simulink model "AutopilotControlSystem"  (R2019b)
settings: configuration reference "ctrlConfigSet" (kept outside this file)
undefined symbols (not defined in the file): ap, DiscIntNeverNeededParam, Earth, env, sensors, uav, WGS84
libraries: mbdriLib x74, simulink x12, aerolibtransform2 x5, simulink_need_slupdate x1, aerolibconvert2 x1
(part 2 of 3)

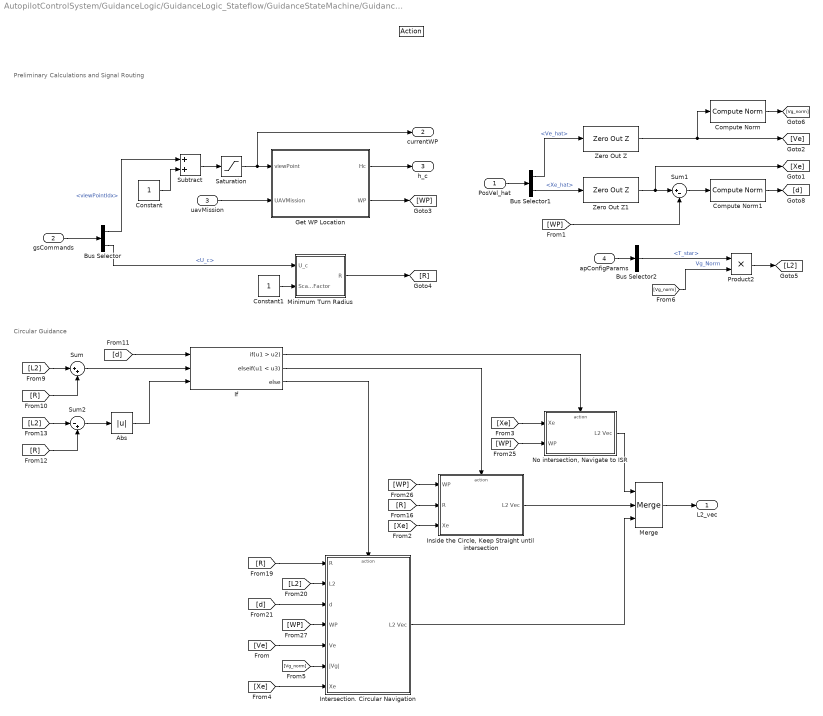
== system AutopilotControlSystem/GuidanceLogic/GuidanceLogic_Stateflow/GuidanceStateMachine/GuidanceLogic.Orbit ==
  note: Preliminary Calculations and Signal Routing
  note: Circular Guidance
  PosVel_hat : Inport
  gsCommands : Inport  Port=2
  uavMission : Inport  Port=3
  apConfigParams : Inport  Port=4
  " " : ActionPort
      settings: CopyFcn=Stateflow.SLINSF.SimulinkMan.removeBlockPreDeleteFcn  PreDeleteFcn=Stateflow.SLINSF.SimulinkMan.unsafePredeleteFcn
  " Compute Norm" : mbdriLib/Utilities/ Compute Norm  SystemSampleTime=-1  Latency=0  AutoFrameSizeCalculation=off
      settings: SourceProductName=Robotics System Toolbox  SourceProductBaseCode=RO
  " Compute Norm1" : mbdriLib/Utilities/ Compute Norm  SystemSampleTime=-1  Latency=0  AutoFrameSizeCalculation=off
      settings: SourceProductName=Robotics System Toolbox  SourceProductBaseCode=RO
  Abs : Abs
  Bus Selector : BusSelector  OutputSignals=viewPointIdx,U_c
  Bus Selector1 : BusSelector  OutputSignals=Ve_hat,Xe_hat
  Bus Selector2 : BusSelector  OutputSignals=T_star
  Constant : Constant  OutDataTypeStr=uint8
      settings: AttributesFormatString=%<Value>
  Constant1 : Constant  OutDataTypeStr=single
      settings: AttributesFormatString=%<Value>
  Get WP Location : Subsystem
  If : If  NumInputs=3  IfExpression=u1 > u2  ElseIfExpressions=u1 < u3
  "Inside the Circle, Keep Straight until intersection" : Subsystem  TreatAsAtomicUnit=on
  Intersection. Circular Navigation : Subsystem  TreatAsAtomicUnit=on
  Merge : Merge  Inputs=3
  Minimum Turn Radius : Subsystem
  "No intersection, Navigate to ISR" : Subsystem  TreatAsAtomicUnit=on
  Product2 : Product
  Saturation : Saturate  UpperLimit=9  LowerLimit=1
      settings: AttributesFormatString=[%<LowerLimit> %<UpperLimit>]
  Subtract : Sum  Inputs=2
  Sum : Sum  Inputs=|++
  Sum1 : Sum  Inputs=|+-
  Sum2 : Sum  Inputs=|-+
  Zero Out Z : mbdriLib/Utilities/Zero Out Z  SystemSampleTime=-1  Latency=0  AutoFrameSizeCalculation=off
      settings: SourceProductName=Robotics System Toolbox  SourceProductBaseCode=RO
  Zero Out Z1 : mbdriLib/Utilities/Zero Out Z  SystemSampleTime=-1  Latency=0  AutoFrameSizeCalculation=off
      settings: SourceProductName=Robotics System Toolbox  SourceProductBaseCode=RO
  L2_vec : Outport  VectorParamsAs1DForOutWhenUnconnected=off
  currentWP : Outport  Port=2  VectorParamsAs1DForOutWhenUnconnected=off
  h_c : Outport  Port=3  VectorParamsAs1DForOutWhenUnconnected=off
  wires:
  [Xe] -> "No intersection, Navigate to ISR"/1(Xe)
  " Compute Norm1"/1 -> [d]
  [WP] -> Intersection. Circular Navigation/4(WP)
  Abs/1 -> If/3
  [Xe] -> Intersection. Circular Navigation/7(Xe)
  Intersection. Circular Navigation/1(L2 Vec) -> Merge/3
  Bus Selector/1 -> Subtract/1  "<viewPointIdx>"
  If/2 -> "Inside the Circle, Keep Straight until intersection"/Action
  [R] -> Intersection. Circular Navigation/1(R)
  "No intersection, Navigate to ISR"/1(L2 Vec) -> Merge/1
  [R] -> Sum2/2
  If/3 -> Intersection. Circular Navigation/Action
  [L2] -> Sum2/1
  "Inside the Circle, Keep Straight until intersection"/1(L2 Vec) -> Merge/2
  uavMission/1 -> Get WP Location/2(UAVMission)
  [Vg_norm] -> Intersection. Circular Navigation/6(|Vg|)
  [Xe] -> "Inside the Circle, Keep Straight until intersection"/3(Xe)
  [WP] -> "No intersection, Navigate to ISR"/2(WP)
  [WP] -> "Inside the Circle, Keep Straight until intersection"/1(WP)
  Get WP Location/2(WP) -> [WP]
  [L2] -> Sum/1
  Subtract/1 -> Saturation/1
  Saturation/1 -> currentWP/1, Get WP Location/1(viewPoint)
  Merge/1 -> L2_vec/1
  Constant/1 -> Subtract/2
  Sum2/1 -> Abs/1
  If/1 -> "No intersection, Navigate to ISR"/Action
  [WP] -> Sum1/2
  [R] -> Sum/2
  [L2] -> Intersection. Circular Navigation/2(L2)
  Sum/1 -> If/2
  [Ve] -> Intersection. Circular Navigation/5(Ve)
  [d] -> If/1
  [R] -> "Inside the Circle, Keep Straight until intersection"/2(R)
  [d] -> Intersection. Circular Navigation/3(d)
  Get WP Location/1(Hc) -> h_c/1
  gsCommands/1 -> Bus Selector/1
  PosVel_hat/1 -> Bus Selector1/1
  Bus Selector1/1 -> Zero Out Z/1  "<Ve_hat>"
  Sum1/1 -> " Compute Norm1"/1
  Zero Out Z/1 -> " Compute Norm"/1, [Ve]
  " Compute Norm"/1 -> [Vg_norm]
  apConfigParams/1 -> Bus Selector2/1
  [Vg_norm] -> Product2/2  "Vg_Norm"
  Product2/1 -> [L2]
  Bus Selector2/1 -> Product2/1  "<T_star>"
  Bus Selector/2 -> Minimum Turn Radius/1(U_c)  "<U_c>"
  Constant1/1 -> Minimum Turn Radius/2(Scale Factor)
  Minimum Turn Radius/1(R) -> [R]
  Zero Out Z1/1 -> Sum1/1, [Xe]
  Bus Selector1/2 -> Zero Out Z1/1  "<Xe_hat>"

== system AutopilotControlSystem/GuidanceLogic/GuidanceLogic_Stateflow/GuidanceStateMachine/GuidanceLogic.RTB ==
  PosVel_hat : Inport
  gsCommands : Inport  Port=2
  uavMission : Inport  Port=3
  " " : ActionPort
      settings: CopyFcn=Stateflow.SLINSF.SimulinkMan.removeBlockPreDeleteFcn  PreDeleteFcn=Stateflow.SLINSF.SimulinkMan.unsafePredeleteFcn
  Bus Selector : BusSelector  OutputSignals=h_c_midLevel,followMobile,MobileLocation
  Bus Selector1 : BusSelector  OutputSignals=Xe_hat
  Constant : Constant  Value=[0 0 0]  OutDataTypeStr=single
      settings: AttributesFormatString=%<Value>
  Get Mobile Location : Subsystem
  RTB1 : Constant  OutDataTypeStr=uint8
      settings: AttributesFormatString=%<Value>
  RTB2 : Constant  OutDataTypeStr=single
      settings: AttributesFormatString=%<Value>
  Simple Predictor : Subsystem
  Slider Gain : simulink/Math Operations/Slider Gain  gain=3  low=1  high=20
  Subtract : Sum  Inputs=+-
  Switch : Switch  Criteria=u2 > Threshold
  Zero Out Z : mbdriLib/Utilities/Zero Out Z  SystemSampleTime=-1  Latency=0  AutoFrameSizeCalculation=off
      settings: SourceProductName=Robotics System Toolbox  SourceProductBaseCode=RO
  L2_vec : Outport  VectorParamsAs1DForOutWhenUnconnected=off
  h_c : Outport  Port=2  VectorParamsAs1DForOutWhenUnconnected=off
  currentWP : Outport  Port=3  VectorParamsAs1DForOutWhenUnconnected=off
  wires:
  gsCommands/1 -> Bus Selector/1
  Bus Selector/3 -> Get Mobile Location/1(Mobile Loc)  "<MobileLocation>"
  Bus Selector/2 -> Get Mobile Location/Enable, Switch/2  "<followMobile>"
  Bus Selector/1 -> h_c/1  "<h_c_midLevel>"
  Simple Predictor/1(Predicted Bp) -> L2_vec/1
  RTB1/1 -> currentWP/1
  PosVel_hat/1 -> Bus Selector1/1
  Bus Selector1/1 -> Zero Out Z/1  "<Xe_hat>"
  Zero Out Z/1 -> Subtract/2
  uavMission/1 -> Get Mobile Location/2(UAVMission)
  Slider Gain/1 -> Simple Predictor/2(Prediction Gain)
  RTB2/1 -> Slider Gain/1
  Switch/1 -> Subtract/1
  Subtract/1 -> Simple Predictor/1(Base Point)
  Get Mobile Location/1(MobileLTP) -> Switch/1
  Constant/1 -> Switch/3

== system AutopilotControlSystem/GuidanceLogic/GuidanceLogic_Stateflow/GuidanceStateMachine/GuidanceLogic.WP ==
  note: Curry, R., Lizarraga, M., Elkaim, G., Mairs, B., “L2+, an Improved Line of Sight Guidance Law for UAVs”
      | American Control Conference, ACC13, Washington D.C., 17-19 June 2013
  PosVel_hat : Inport
  gsCommands : Inport  Port=2
  uavMission : Inport  Port=3
  apConfigParams : Inport  Port=4
  " " : ActionPort
      settings: CopyFcn=Stateflow.SLINSF.SimulinkMan.removeBlockPreDeleteFcn  PreDeleteFcn=Stateflow.SLINSF.SimulinkMan.unsafePredeleteFcn
  Bus Selector : BusSelector  OutputSignals=isManualModeOn
  Bus Selector1 : BusSelector  OutputSignals=Ve_hat,Xe_hat
  Bus Selector2 : BusSelector  OutputSignals=T_star,turnLead
  Compute Distance to WP : Subsystem
  Compute L2 Vector : Subsystem
  Compute Vg_norm : Subsystem
  Delay : Delay  DelayLength=1  InitialCondition=1000
  Display : Display
  Get Next Waypoint : Subsystem
  Logical Operator : Logic  Operator=NOT  AllPortsSameDT=off  OutDataTypeStr=boolean
  MATLAB Function : MATLAB Function  TreatAsAtomicUnit=on
  Product1 : Product  OutDataTypeStr=single  RndMeth=Zero
  Product2 : Product
  Recent Enable : Subsystem
  Subtract : Sum  Inputs=+-
  Wp Switching Logic : mbdriLib/Guidance/Wp Switching Logic  SystemSampleTime=-1  Latency=0  AutoFrameSizeCalculation=off
      settings: SourceProductName=Robotics System Toolbox  SourceProductBaseCode=RO
  L2_vec : Outport  VectorParamsAs1DForOutWhenUnconnected=off
  currentWP : Outport  Port=2  VectorParamsAs1DForOutWhenUnconnected=off
  h_c : Outport  Port=3  VectorParamsAs1DForOutWhenUnconnected=off
  wires:
  Recent Enable/1(WPEnable) -> Wp Switching Logic/3
  uavMission/1 -> MATLAB Function/1(u), Get Next Waypoint/1(UAVMission)
  Wp Switching Logic/1 -> Get Next Waypoint/2(From WP)
  Subtract/1 -> Delay/1
  Delay/1 -> Wp Switching Logic/1
  Compute Distance to WP/1(Dist2WpT) -> Subtract/1, Compute L2 Vector/1(Dist2WP)
  Product1/1 -> Subtract/2  "turnLeadDistance"
  [Xe] -> Compute L2 Vector/5(Xe)
  Get Next Waypoint/1(H_c) -> h_c/1
  Compute L2 Vector/1(L2Vec) -> L2_vec/1
  Get Next Waypoint/3(T) -> Compute L2 Vector/3(T), Compute Distance to WP/3(T)
  Product2/1 -> Get Next Waypoint/4(L2), Compute L2 Vector/6(L2)
  Get Next Waypoint/2(WPT) -> Compute L2 Vector/2(WPT), Compute Distance to WP/2(WPT)
  Get Next Waypoint/4(N) -> Compute L2 Vector/4(N)
  MATLAB Function/1(maxWp) -> Wp Switching Logic/2
  Wp Switching Logic/2 -> currentWP/1, Get Next Waypoint/3(To WP)
  gsCommands/1 -> Bus Selector/1
  Logical Operator/1 -> Recent Enable/1(WP Fly)
  Bus Selector/1 -> Logical Operator/1  "<isManualModeOn>"
  PosVel_hat/1 -> Bus Selector1/1
  Bus Selector1/2 -> Display/1, [Xe], Compute Distance to WP/1(Xe)  "<Xe_hat>"
  [Vg_norm] -> Product2/2  "Vg_Norm"
  apConfigParams/1 -> Bus Selector2/1
  Compute Vg_norm/1(|Vg|) -> [Vg_norm], Product1/2
  Bus Selector1/1 -> Compute Vg_norm/1(<Ve_hat>)  "<Ve_hat>"
  [turnLead] -> Product1/1
  Bus Selector2/1 -> Product2/1  "<T_star>"
  Bus Selector2/2 -> [turnLead]  "<turnLead>"

== system AutopilotControlSystem/InnerLoopAutopilot/Latch Trim Conditions/Latch Control Surfaces Trim from any mode ==
  ctrlSurfaces : Inport
  Trigger : TriggerPort  TriggerType=falling  VariantControl=Variant
  Trim : Outport  VectorParamsAs1DForOutWhenUnconnected=off
  wires:
  ctrlSurfaces/1 -> Trim/1

== system AutopilotControlSystem/InnerLoopAutopilot/Longitudinal Channel/Compute Feed Forward ==
  dEFFGain : Inport
  SensorData : Inport  Port=2
  1D Discrete Filter : mbdriLib/Filtering/1D Discrete Filter  bw=10  TSample=ap.apSampleTime
      settings: AttributesFormatString=Fc = 10  SourceProductName=Robotics System Toolbox  SourceProductBaseCode=RO
  Add5 : Sum  Inputs=+-  OutDataTypeStr=single
  Bus Selector : BusSelector  OutputSignals=Euler
  Constant2 : Constant  OutDataTypeStr=single
      settings: AttributesFormatString=%<Value>
  Constant4 : Constant  OutDataTypeStr=single
      settings: AttributesFormatString=%<Value>
  Product : Product  Inputs=*/  RndMeth=Zero
  Product1 : Product  RndMeth=Zero
  Selector : Selector  InputPortWidth=3  IndexOptions=Index vector (dialog)  Indices=[1]  OutputSizes=1
  Trigonometric Function : Trigonometry  Operator=cos
  "[-60 60]" : Saturate  UpperLimit=60  LowerLimit=-60
      settings: AttributesFormatString="[%<LowerLimit>  %<UpperLimit>]"
  FF : Outport  VectorParamsAs1DForOutWhenUnconnected=off
  wires:
  Selector/1 -> 1D Discrete Filter/1
  Product/1 -> Add5/1
  Constant4/1 -> Product/1
  1D Discrete Filter/1 -> "[-60 60]"/1
  Trigonometric Function/1 -> Product/2
  Constant2/1 -> Add5/2
  Product1/1 -> FF/1
  Add5/1 -> Product1/2
  "[-60 60]"/1 -> Trigonometric Function/1
  Bus Selector/1 -> Selector/1  "<Euler>"
  dEFFGain/1 -> Product1/1
  SensorData/1 -> Bus Selector/1

== system AutopilotControlSystem/InnerLoopAutopilot/Longitudinal Channel/Height Error to Pitch Command [PI] ==
  Error : Inport
  Reset : Inport  Port=2
  PIDGains : Inport  Port=3
  Demux : Demux  Outputs=3
  PID Controller : simulink/Continuous/PID Controller  Controller=PI  Form=Parallel  TimeDomain=Discrete-time  SampleTime=ap.apSampleTime  IntegratorMethod=Trapezoidal  FilterMethod=Forward Euler  ControllerParametersSource=external  P=1  I=1  D=0  UseFilter=on  N=100  TunerSelectOption=Transfer Function Based (PID Tuner App)  InitialConditionSource=internal  InitialConditionForIntegrator=0  InitialConditionForFilter=0  DifferentiatorICPrevScaledInput=0  ExternalReset=level  TrackingMode=off  Kt=1  LimitOutput=on  UpperSaturationLimit=ap.control.the_cLimit  LowerSaturationLimit=-ap.control.the_cLimit  LinearizeAsGain=on  AntiWindupMode=clamping  Kb=1  POutMin=[]  POutMax=[]  IOutMin=[]  IOutMax=[]  DOutMin=[]  DOutMax=[]  NOutMin=[]  NOutMax=[]  SumOutMin=[]  SumOutMax=[]  SaturationOutMin=[]  SaturationOutMax=[]  PParamMin=[]  PParamMax=[]  IParamMin=[]  IParamMax=[]  DParamMin=[]  DParamMax=[]  NParamMin=[]  NParamMax=[]  KbParamMin=[]  KbParamMax=[]  KtParamMin=[]  KtParamMax=[]  KbOutMin=[]  KbOutMax=[]  KtOutMin=[]  KtOutMax=[]  IntegratorOutMin=[]  IntegratorOutMax=[]  FilterOutMin=[]  FilterOutMax=[]  SumI1OutMin=[]  SumI1OutMax=[]  SumI2OutMin=[]  SumI2OutMax=[]  SumI3OutMin=[]  SumI3OutMax=[]  SumI4OutMin=[]  SumI4OutMax=[]  SumDOutMin=[]  SumDOutMax=[]  DifferentiatorOutMin=[]  DifferentiatorOutMax=[]  FilterDiffOutCoefMin=[]  FilterDiffOutCoefMax=[]  ReciprocalOutMin=[]  ReciprocalOutMax=[]  SumDenOutMin=[]  SumDenOutMax=[]  SumNumOutMin=[]  SumNumOutMax=[]  DivideOutMin=[]  DivideOutMax=[]  IntegratorContinuousStateAttributes=''  IntegratorStateMustResolveToSignalObject=off  IntegratorRTWStateStorageClass=Auto  FilterContinuousStateAttributes=''  FilterStateMustResolveToSignalObject=off  FilterRTWStateStorageClass=Auto  ParallelPVariant=ExternalParameters  IdealPVariant=Disabled  IVariant=ExternalParameters  DVariant=Disabled  IntegratorVariant=Discrete  SatVariant=Enabled  AWVariant=DiscClampingParallel  PCopyVariant=Disabled  TRVariant=Disabled  FdbkBlocksVariant=Feedback  IdealPFdbkVariant=Passthrough  SatFdbkVariant=Passthrough  DerivativeFilterVariant=Disabled  NVariant=Disabled  NCopyVariant=Disabled_SignalSpec  FilterICVariant=Disabled  IntegratorICVariant=InternalICs  ExternalResetVariant=ExternalReset  TRSumVariant=Passthrough  SumFdbkVariant=Enabled  SumVariant=Sum_PI
  Terminator : Terminator
  Output : Outport  VectorParamsAs1DForOutWhenUnconnected=off
  wires:
  Demux/3 -> Terminator/1
  Error/1 -> PID Controller/1
  PIDGains/1 -> Demux/1
  Demux/1 -> PID Controller/2
  Demux/2 -> PID Controller/3
  Reset/1 -> PID Controller/4
  PID Controller/1 -> Output/1

== system AutopilotControlSystem/InnerLoopAutopilot/Longitudinal Channel/Rate Limiter Dynamic with External IC and Autoreset for Change in IC ==
  note: Y(k)
  note: U(k)
  up : Inport
  u : Inport  Port=2
  IC : Inport  Port=3
  lo : Inport  Port=4
  Capture/Reset IC : Subsystem
  Difference Inputs1 : Sum  Description=Add in CPU  DisableCoverage=on  Inputs=+-  OutDataTypeStr=Inherit: Inherit via back propagation
  Difference Inputs2 : Sum  Description=Add in CPU  OutDataTypeStr=Inherit: Inherit via back propagation
  FixPt Data Type Duplicate : DataTypeDuplicate  DisableCoverage=on  NumInputPorts=7
  Saturation Dynamic : simulink/Discontinuities/Saturation Dynamic  OutMin=[]  OutMax=[]  OutDataTypeStr=Inherit: Same as second input  OutDataType=fixdt(1, 16)  OutScaling=2^-10  DoSatur=off
  delta fall limit : Product  DisableCoverage=on  Inputs=**  OutDataTypeStr=Inherit: Inherit via back propagation  SaturateOnIntegerOverflow=on
  delta rise limit : Product  DisableCoverage=on  Inputs=**  OutDataTypeStr=Inherit: Inherit via back propagation  SaturateOnIntegerOverflow=on
  sample time : SampleTimeMath  DisableCoverage=on  TsampMathOp=Ts Only  weightValue=1
  Y : Outport  VectorParamsAs1DForOutWhenUnconnected=off
  wires:
  sample time/1 -> delta fall limit/2, delta rise limit/2
  lo/1 -> delta fall limit/1
  delta rise limit/1 -> FixPt Data Type Duplicate/6, Saturation Dynamic/1
  up/1 -> delta rise limit/1
  Difference Inputs2/1 -> FixPt Data Type Duplicate/1, Capture/Reset IC/1(Y(k)), Y/1
  Saturation Dynamic/1 -> Difference Inputs2/1, FixPt Data Type Duplicate/7
  delta fall limit/1 -> FixPt Data Type Duplicate/3, Saturation Dynamic/3
  u/1 -> Difference Inputs1/1, FixPt Data Type Duplicate/5, sample time/1
  Difference Inputs1/1 -> FixPt Data Type Duplicate/4, Saturation Dynamic/2  "( U(k) - Y(k-1) )"
  Capture/Reset IC/1(Y(k-1)) -> Difference Inputs2/2, FixPt Data Type Duplicate/2, Difference Inputs1/2
  IC/1 -> Capture/Reset IC/2(IC)

== system AutopilotControlSystem/Navigation Filter/Get Vn Ve/Subsystem5 ==
  u : Inport
  Trigonometric Function : Trigonometry
  Trigonometric Function1 : Trigonometry  Operator=cos
  sin(u) : Outport  VectorParamsAs1DForOutWhenUnconnected=off
  cos(u) : Outport  Port=2  VectorParamsAs1DForOutWhenUnconnected=off
  wires:
  u/1 -> Trigonometric Function/1, Trigonometric Function1/1
  Trigonometric Function/1 -> sin(u)/1
  Trigonometric Function1/1 -> cos(u)/1

== system AutopilotControlSystem/Navigation Filter/Position&Velocity Filter/CompRateOnly ==
  LoPass : Inport
  Gain : Gain  Gain=omega
      settings: AttributesFormatString=%<Gain>
  Sum1 : Sum  Inputs=|+-
  Unit Delay : UnitDelay  SampleTime=T  HasFrameUpgradeWarning=on
  ZPK 1D Discrete Filter : mbdriLib/Filtering/ZPK 1D Discrete Filter  zval=[]  pval=[0]  kval=1  TSample=0.01
      settings: SourceProductName=Robotics System Toolbox  SourceProductBaseCode=RO
  Rate_hat : Outport  VectorParamsAs1DForOutWhenUnconnected=off
  wires:
  Unit Delay/1 -> Sum1/2
  LoPass/1 -> Sum1/1
  Sum1/1 -> Gain/1
  Gain/1 -> ZPK 1D Discrete Filter/1, Rate_hat/1
  ZPK 1D Discrete Filter/1 -> Unit Delay/1

== system AutopilotControlSystem/Navigation Filter/Position&Velocity Filter/Deriv  ==
  y : Inport
  Gain2 : Gain  Gain=[ 1/(5*ap.apSampleTime) ]
      settings: AttributesFormatString=%<Gain>
  Integer Delay1 : Delay  DelayLength=5  InitialCondition=0  SampleTime=ap.apSampleTime
  Sum5 : Sum  Inputs=-+|
  ydot : Outport  VectorParamsAs1DForOutWhenUnconnected=off
  wires:
  Gain2/1 -> ydot/1
  y/1 -> Integer Delay1/1, Sum5/2
  Integer Delay1/1 -> Sum5/1
  Sum5/1 -> Gain2/1

== system AutopilotControlSystem/Navigation Filter/Position&Velocity Filter/VN Ve Filter ==
  Vn : Inport
  Ve : Inport  Port=2
  New GPS : Inport  Port=3
  Enable : EnablePort
  Constant : Constant  Value=ap.apSampleTime
      settings: AttributesFormatString=%<Value>
  RateAid for GPS : mbdriLib/Filtering/RateAid for GPS  SystemSampleTime=-1  Latency=0  AutoFrameSizeCalculation=off
      settings: SourceProductName=Robotics System Toolbox  SourceProductBaseCode=RO
  RateAid for GPS1 : mbdriLib/Filtering/RateAid for GPS  SystemSampleTime=-1  Latency=0  AutoFrameSizeCalculation=off
      settings: SourceProductName=Robotics System Toolbox  SourceProductBaseCode=RO
  Vn_fil : Outport  OutputWhenDisabled=reset  InitialOutput=0  VectorParamsAs1DForOutWhenUnconnected=off
  Ve_fil : Outport  Port=2  OutputWhenDisabled=reset  InitialOutput=0  VectorParamsAs1DForOutWhenUnconnected=off
  wires:
  Constant/1 -> RateAid for GPS1/3, RateAid for GPS/3
  New GPS/1 -> RateAid for GPS/2, RateAid for GPS1/2
  Vn/1 -> RateAid for GPS/1
  Ve/1 -> RateAid for GPS1/1
  RateAid for GPS/1 -> Vn_fil/1
  RateAid for GPS1/1 -> Ve_fil/1

== system AutopilotControlSystem/Navigation Filter/Position&Velocity Filter/Z Comp Filter ==
  note: Lizarraga, Mariano I. Autonomous landing system for a UAV . Master's Thesis. Monterey California. Naval Postgraduate School, 2004.
  Az : Inport
  Baro Alt : Inport  Port=2
  Xe_z_ic : Inport  Port=3
  Constant : Constant  Value=env.ISA_g  OutDataTypeStr=single
      settings: AttributesFormatString=%<Value>
  Discrete-Time Integrator : DiscreteIntegrator  gainval=1  SampleTime=-1  ICPrevOutput=DiscIntNeverNeededParam  ICPrevScaledInput=DiscIntNeverNeededParam
  Discrete-Time Integrator1 : DiscreteIntegrator  gainval=1  SampleTime=-1  ICPrevOutput=DiscIntNeverNeededParam  ICPrevScaledInput=DiscIntNeverNeededParam
  Discrete-Time Integrator2 : DiscreteIntegrator  gainval=1  InitialConditionSource=external  SampleTime=-1  ICPrevOutput=DiscIntNeverNeededParam  ICPrevScaledInput=DiscIntNeverNeededParam
  Gain : Gain  Gain=21  OutDataTypeStr=single
      settings: AttributesFormatString=%<Gain>
  Gain1 : Gain  Gain=9  OutDataTypeStr=single
      settings: AttributesFormatString=%<Gain>
  Gain2 : Gain  Gain=15  OutDataTypeStr=single
      settings: AttributesFormatString=%<Gain>
  Sum : Sum  Inputs=|++
  Sum1 : Sum  Inputs=+++
  Sum2 : Sum  Inputs=-+|
  Sum3 : Sum  Inputs=|++
  Xe_Z_hat : Outport  VectorParamsAs1DForOutWhenUnconnected=off
  wires:
  Discrete-Time Integrator2/1 -> Sum2/1, Xe_Z_hat/1
  Gain2/1 -> Sum3/2
  Gain1/1 -> Discrete-Time Integrator/1
  Gain/1 -> Sum1/3
  Sum2/1 -> Gain2/1, Gain/1, Gain1/1
  Sum3/1 -> Discrete-Time Integrator2/1
  Discrete-Time Integrator1/1 -> Sum3/1
  Baro Alt/1 -> Sum2/2
  Xe_z_ic/1 -> Discrete-Time Integrator2/2
  Sum1/1 -> Discrete-Time Integrator1/1
  Sum/1 -> Sum1/1
  Discrete-Time Integrator/1 -> Sum1/2
  Constant/1 -> Sum/2
  Az/1 -> Sum/1

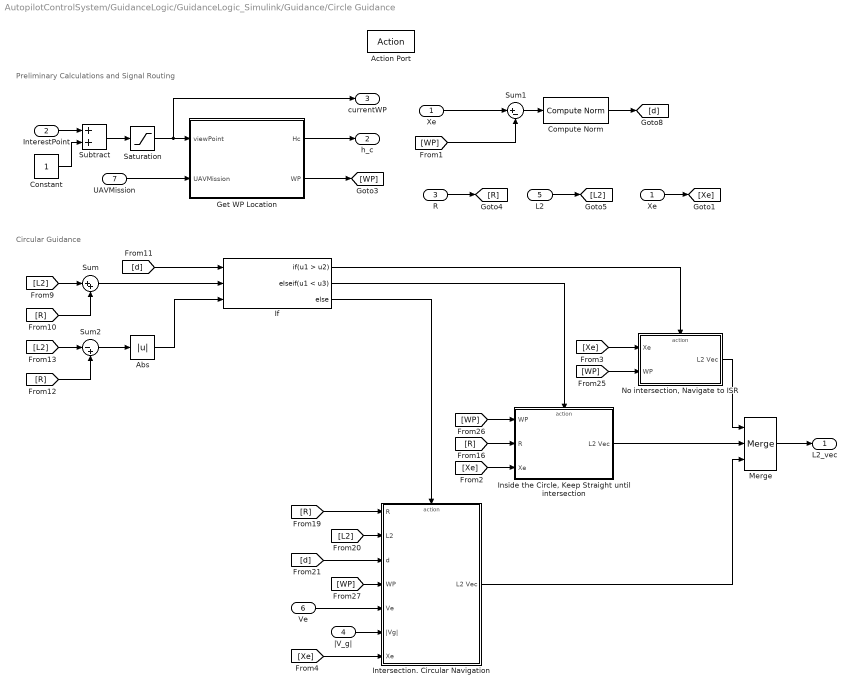
== system AutopilotControlSystem/GuidanceLogic/GuidanceLogic_Simulink/Guidance/Circle Guidance ==
  note: Preliminary Calculations and Signal Routing
  note: Circular Guidance
  Xe : Inport
  InterestPoint : Inport  Port=2
  R : Inport  Port=3
  |V_g| : Inport  Port=4
  L2 : Inport  Port=5
  Ve : Inport  Port=6
  UAVMission : Inport  Port=7
  Action Port : ActionPort  ActionPortLabel=elseif { }
  " Compute Norm" : mbdriLib/Utilities/ Compute Norm
      settings: SourceProductName=Robotics System Toolbox  SourceProductBaseCode=RO
  Abs : Abs
  Constant : Constant  OutDataTypeStr=uint8
      settings: AttributesFormatString=%<Value>
  Get WP Location : Subsystem
  If : If  NumInputs=3  IfExpression=u1 > u2  ElseIfExpressions=u1 < u3
  "Inside the Circle, Keep Straight until intersection" : Subsystem  TreatAsAtomicUnit=on
  Intersection. Circular Navigation : Subsystem  TreatAsAtomicUnit=on
  Merge : Merge  Inputs=3
  "No intersection, Navigate to ISR" : Subsystem  TreatAsAtomicUnit=on
  Saturation : Saturate  UpperLimit=9  LowerLimit=1
      settings: AttributesFormatString=[%<LowerLimit> %<UpperLimit>]
  Subtract : Sum  Inputs=2
  Sum : Sum  Inputs=|++
  Sum1 : Sum  Inputs=|+-
  Sum2 : Sum  Inputs=|-+
  "Xe   " : InportShadow
  L2_vec : Outport  VectorParamsAs1DForOutWhenUnconnected=off
  h_c : Outport  Port=2  VectorParamsAs1DForOutWhenUnconnected=off
  currentWP : Outport  Port=3  VectorParamsAs1DForOutWhenUnconnected=off
  wires:
  Saturation/1 -> Get WP Location/1(viewPoint), currentWP/1
  InterestPoint/1 -> Subtract/1
  Subtract/1 -> Saturation/1
  Constant/1 -> Subtract/2
  [Xe] -> "No intersection, Navigate to ISR"/1(Xe)
  [Xe] -> "Inside the Circle, Keep Straight until intersection"/3(Xe)
  Xe/1 -> [Xe]
  Intersection. Circular Navigation/1(L2 Vec) -> Merge/3
  "Inside the Circle, Keep Straight until intersection"/1(L2 Vec) -> Merge/2
  "No intersection, Navigate to ISR"/1(L2 Vec) -> Merge/1
  UAVMission/1 -> Get WP Location/2(UAVMission)
  R/1 -> [R]
  Get WP Location/2(WP) -> [WP]
  L2/1 -> [L2]
  [L2] -> Sum/1
  [R] -> Sum/2
  "Xe   "/1 -> Sum1/1
  [WP] -> Sum1/2
  Sum1/1 -> " Compute Norm"/1
  " Compute Norm"/1 -> [d]
  [d] -> If/1
  Sum/1 -> If/2
  [L2] -> Sum2/1
  [R] -> Sum2/2
  Sum2/1 -> Abs/1
  Abs/1 -> If/3
  Merge/1 -> L2_vec/1
  If/1 -> "No intersection, Navigate to ISR"/Action
  If/2 -> "Inside the Circle, Keep Straight until intersection"/Action
  If/3 -> Intersection. Circular Navigation/Action
  [WP] -> "No intersection, Navigate to ISR"/2(WP)
  [WP] -> "Inside the Circle, Keep Straight until intersection"/1(WP)
  [R] -> "Inside the Circle, Keep Straight until intersection"/2(R)
  [R] -> Intersection. Circular Navigation/1(R)
  [L2] -> Intersection. Circular Navigation/2(L2)
  [d] -> Intersection. Circular Navigation/3(d)
  [WP] -> Intersection. Circular Navigation/4(WP)
  Ve/1 -> Intersection. Circular Navigation/5(Ve)
  |V_g|/1 -> Intersection. Circular Navigation/6(|Vg|)
  Get WP Location/1(Hc) -> h_c/1
  [Xe] -> Intersection. Circular Navigation/7(Xe)

== system AutopilotControlSystem/GuidanceLogic/GuidanceLogic_Simulink/Guidance/Mid Level Direct Commands ==
  psiDot_c_ml : Inport
  h_c_midLvl : Inport  Port=2
  U_m : Inport  Port=3
  Action Port : ActionPort  ActionPortLabel=elseif { }
  RTB1 : Constant  Value=0  OutDataTypeStr=uint8
      settings: AttributesFormatString=%<Value>
  psi_dot to phi : mbdriLib/Angles and Units/psi_dot to phi
      settings: SourceProductName=Robotics System Toolbox  SourceProductBaseCode=RO
  phi_c_ml : Outport  VectorParamsAs1DForOutWhenUnconnected=off
  h_c : Outport  Port=2  VectorParamsAs1DForOutWhenUnconnected=off
  currentWP : Outport  Port=3  VectorParamsAs1DForOutWhenUnconnected=off
  wires:
  RTB1/1 -> currentWP/1
  psi_dot to phi/1 -> phi_c_ml/1
  psiDot_c_ml/1 -> psi_dot to phi/1
  U_m/1 -> psi_dot to phi/2
  h_c_midLvl/1 -> h_c/1

== system AutopilotControlSystem/GuidanceLogic/GuidanceLogic_Simulink/Guidance/Minimum Turn Radius ==
  U_c : Inport
  Scale Factor : Inport  Port=2
  Constant1 : Constant  Value=ap.guidance.maxAcc  OutDataTypeStr=single
      settings: AttributesFormatString=%<Value>
  IC : InitialCondition  Value=1.5
  Math Function : Math  Operator=square  SaturateOnIntegerOverflow=on
  Product2 : Product  RndMeth=Zero
  Product3 : Product  Inputs=*/  RndMeth=Zero
  "[1.5 10]" : Saturate  UpperLimit=10  LowerLimit=1.5
      settings: AttributesFormatString="[%<LowerLimit>  %<UpperLimit>]"
  R : Outport  VectorParamsAs1DForOutWhenUnconnected=off
  wires:
  IC/1 -> "[1.5 10]"/1
  "[1.5 10]"/1 -> Product2/1
  Product3/1 -> R/1
  Scale Factor/1 -> IC/1
  Math Function/1 -> Product2/2
  Constant1/1 -> Product3/2
  Product2/1 -> Product3/1
  U_c/1 -> Math Function/1

== system AutopilotControlSystem/GuidanceLogic/GuidanceLogic_Simulink/Guidance/RTB//Follow Mobile Guidance ==
  Mobile Location : Inport
  Follow Mobile? : Inport  Port=2
  MidLvl h_c : Inport  Port=3
  Puav : Inport  Port=4
  UAVMission : Inport  Port=5
  Action Port : ActionPort  ActionPortLabel=if { }
  Constant : Constant  Value=[0 0 0]  OutDataTypeStr=single
      settings: AttributesFormatString=%<Value>
  Get Mobile Location : Subsystem
  RTB1 : Constant  OutDataTypeStr=uint8
      settings: AttributesFormatString=%<Value>
  RTB2 : Constant  OutDataTypeStr=single
      settings: AttributesFormatString=%<Value>
  Simple Predictor : Subsystem
  Slider Gain : simulink/Math Operations/Slider Gain  gain=3  low=1  high=20
  Subtract : Sum  Inputs=+-
  Switch : Switch  Criteria=u2 > Threshold
  L2_vec : Outport  VectorParamsAs1DForOutWhenUnconnected=off
  h_c : Outport  Port=2  VectorParamsAs1DForOutWhenUnconnected=off
  currentWP : Outport  Port=3  VectorParamsAs1DForOutWhenUnconnected=off
  wires:
  RTB1/1 -> currentWP/1
  UAVMission/1 -> Get Mobile Location/2(UAVMission)
  Slider Gain/1 -> Simple Predictor/2(Prediction Gain)
  RTB2/1 -> Slider Gain/1
  MidLvl h_c/1 -> h_c/1
  Switch/1 -> Subtract/1
  Puav/1 -> Subtract/2
  Subtract/1 -> Simple Predictor/1(Base Point)
  Simple Predictor/1(Predicted Bp) -> L2_vec/1
  Mobile Location/1 -> Get Mobile Location/1(Mobile Loc)
  Follow Mobile?/1 -> Get Mobile Location/Enable, Switch/2
  Get Mobile Location/1(MobileLTP) -> Switch/1
  Constant/1 -> Switch/3

== system AutopilotControlSystem/GuidanceLogic/GuidanceLogic_Simulink/Guidance/Recent Enable ==
  WP Fly : Inport
  IC1 : InitialCondition  Value=0
  Subsystem : Subsystem
  WPEnable : Outport  VectorParamsAs1DForOutWhenUnconnected=off
  wires:
  WP Fly/1 -> IC1/1
  Subsystem/1(Just Enab) -> WPEnable/1
  IC1/1 -> Subsystem/1(WP Fly)

== system AutopilotControlSystem/GuidanceLogic/GuidanceLogic_Simulink/Guidance/WP Guidance ==
  note: Curry, R., Lizarraga, M., Elkaim, G., Mairs, B., “L2+, an Improved Line of Sight Guidance Law for UAVs”
      | American Control Conference, ACC13, Washington D.C., 17-19 June 2013
  UAVMission : Inport
  Xe : Inport  Port=2
  L2 : Inport  Port=3
  MaxWP : Inport  Port=4
  turnLeadTime : Inport  Port=5
  V_g : Inport  Port=6
  WpEnable : Inport  Port=7
  Action Port : ActionPort  ActionPortLabel=elseif { }
  Compute Distance to WP : Subsystem
  Compute L2 Vector : Subsystem
  Delay : Delay  DelayLength=1  InitialCondition=1000
  Get Next Waypoint : Subsystem
  Product1 : Product  OutDataTypeStr=single  RndMeth=Zero
  Subtract : Sum  Inputs=+-
  Wp Switching Logic : mbdriLib/Guidance/Wp Switching Logic  SystemSampleTime=-1
      settings: SourceProductName=Robotics System Toolbox  SourceProductBaseCode=RO
  L2Vec : Outport  VectorParamsAs1DForOutWhenUnconnected=off
  h_c : Outport  Port=2  VectorParamsAs1DForOutWhenUnconnected=off
  currentWP : Outport  Port=3  VectorParamsAs1DForOutWhenUnconnected=off
  wires:
  Get Next Waypoint/1(H_c) -> h_c/1
  WpEnable/1 -> Wp Switching Logic/3
  Product1/1 -> Subtract/2  "turnLeadDistance"
  turnLeadTime/1 -> Product1/1
  V_g/1 -> Product1/2
  Compute L2 Vector/1(L2Vec) -> L2Vec/1
  MaxWP/1 -> Wp Switching Logic/2
  Subtract/1 -> Delay/1
  L2/1 -> Compute L2 Vector/6(L2), Get Next Waypoint/4(L2)
  Delay/1 -> Wp Switching Logic/1
  [Xe] -> Compute L2 Vector/5(Xe)
  Get Next Waypoint/4(N) -> Compute L2 Vector/4(N)
  Compute Distance to WP/1(Dist2WpT) -> Compute L2 Vector/1(Dist2WP), Subtract/1
  Xe/1 -> Compute Distance to WP/1(Xe), [Xe]
  Get Next Waypoint/3(T) -> Compute Distance to WP/3(T), Compute L2 Vector/3(T)
  Get Next Waypoint/2(WPT) -> Compute Distance to WP/2(WPT), Compute L2 Vector/2(WPT)
  UAVMission/1 -> Get Next Waypoint/1(UAVMission)
  Wp Switching Logic/2 -> Get Next Waypoint/3(To WP), currentWP/1
  Wp Switching Logic/1 -> Get Next Waypoint/2(From WP)

== system AutopilotControlSystem/GuidanceLogic/GuidanceLogic_Stateflow/GuidanceStateMachine/GuidanceLogic.Orbit/Get WP Location ==
  viewPoint : Inport
  UAVMission : Inport  Port=2
  Bus Selector : BusSelector  OutputSignals=wpPos
  Bus Selector1 : BusSelector  OutputSignals=wpPos
  Demux : Demux  Outputs=[2 1]
  Integer Delay1 : Delay  DelayLength=1
  LLA to Flat Earth : aerolibtransform2/LLA to Flat Earth  Commented=on  units=Metric (MKS)  ptype=Earth (WGS84)  F=1/298.257223563  R=6378137  LL0=[0 10]  psi=0
      settings: SourceProductName=Aerospace Blockset  SourceProductBaseCode=AE
  LLA to Flat Earth with Init Pos : mbdriLib/Coordinates/LLA to Flat Earth with Init Pos  R=6378137  F=1/298.2572235  psi=0
      settings: SourceProductName=Robotics System Toolbox  SourceProductBaseCode=RO
  Selector : Selector  InputPortWidth=3  IndexOptions=Index vector (dialog)  Indices=[3]  OutputSizes=1
  Selector1 : Selector  InputPortWidth=10  IndexOptions=Index vector (port)  Indices=[3]  OutputSizes=1
  Selector2 : Selector  InputPortWidth=10  IndexOptions=Index vector (dialog)  Indices=[1]  OutputSizes=1
  Selector3 : Selector  InputPortWidth=3  IndexOptions=Index vector (dialog)  Indices=[3]  OutputSizes=1
  Selector4 : Selector  InputPortWidth=3  IndexOptions=Index vector (dialog)  Indices=[1 2]  OutputSizes=1
  Zero Out Z : mbdriLib/Utilities/Zero Out Z  SystemSampleTime=-1  Latency=0  AutoFrameSizeCalculation=off
      settings: SourceProductName=Robotics System Toolbox  SourceProductBaseCode=RO
  Hc : Outport  VectorParamsAs1DForOutWhenUnconnected=off
  WP : Outport  Port=2  VectorParamsAs1DForOutWhenUnconnected=off
  wires:
  Bus Selector1/1 -> Selector3/1, Selector4/1  "<wpPos>"
  Selector/1 -> Integer Delay1/1
  Integer Delay1/1 -> Hc/1
  UAVMission/1 -> Selector2/1, Selector1/1
  viewPoint/1 -> Selector1/2
  Selector1/1 -> Bus Selector/1
  Bus Selector/1 -> Demux/1  "<wpPos>"
  Demux/2 -> LLA to Flat Earth with Init Pos/2
  Demux/1 -> LLA to Flat Earth with Init Pos/1
  Selector3/1 -> LLA to Flat Earth with Init Pos/3
  Selector2/1 -> Bus Selector1/1
  Selector4/1 -> LLA to Flat Earth with Init Pos/4
  LLA to Flat Earth with Init Pos/1 -> Zero Out Z/1, Selector/1
  Zero Out Z/1 -> WP/1

== system AutopilotControlSystem/GuidanceLogic/GuidanceLogic_Stateflow/GuidanceStateMachine/GuidanceLogic.Orbit/Inside the Circle, Keep Straight until intersection ==
  note: % Compute the top coordinate of the circle
      | % using the circle's parametric equations:
      | % x = a + r cos (t)
      | % y = b + r sin (t)
      | %
      | % @ t =0
  WP : Inport
  R : Inport  Port=2
  Xe : Inport  Port=3
  Action Port : ActionPort  ActionPortLabel=elseif(u1 < u3)
  Demux : Demux  Outputs=[1 2]
  Mux : Mux  Inputs=2
  Subtract : Sum  Inputs=+-  OutDataTypeStr=single
  Subtract1 : Sum  OutDataTypeStr=single
  L2 Vec : Outport  VectorParamsAs1DForOutWhenUnconnected=off
  wires:
  Subtract/1 -> L2 Vec/1
  Xe/1 -> Subtract/2
  Demux/1 -> Subtract1/2
  Subtract1/1 -> Mux/1
  Demux/2 -> Mux/2
  R/1 -> Subtract1/1
  WP/1 -> Demux/1
  Mux/1 -> Subtract/1

== system AutopilotControlSystem/GuidanceLogic/GuidanceLogic_Stateflow/GuidanceStateMachine/GuidanceLogic.Orbit/Intersection. Circular Navigation ==
  R : Inport
  L2 : Inport  Port=2
  d : Inport  Port=3
  WP : Inport  Port=4
  Ve : Inport  Port=5
  |Vg| : Inport  Port=6
  Xe : Inport  Port=7
  Action Port : ActionPort  ActionPortLabel=else
  Compute Hyp : Subsystem
  Compute L2 : Subsystem
  Compute P2 : Subsystem
  Compute the Intersection Points : MATLAB Function  TreatAsAtomicUnit=on
  Product5 : Product  RndMeth=Zero
  Xe1 : InportShadow  Port=7
  "d " : InportShadow  Port=3
  L2 Vec : Outport  VectorParamsAs1DForOutWhenUnconnected=off
  wires:
  Product5/1 -> Compute the Intersection Points/1(hFact)
  R/1 -> Compute Hyp/1(R)
  L2/1 -> Compute Hyp/2(L2)
  d/1 -> Compute Hyp/3(d)
  Compute Hyp/1(h) -> Product5/1
  Compute Hyp/2(a) -> Compute P2/1(a)
  "d "/1 -> Compute P2/2(d)
  WP/1 -> Compute P2/3(WP)
  Xe1/1 -> Compute P2/4(Xe)
  Compute P2/1((Xe-Wp)*d^-1) -> Product5/2
  Compute P2/2(P2) -> Compute the Intersection Points/2(P2)
  Ve/1 -> Compute L2/1(Ve)
  |Vg|/1 -> Compute L2/2(|Vg|)
  Compute the Intersection Points/1(P31) -> Compute L2/3(P31)
  Xe/1 -> Compute L2/4(Xe)
  Compute the Intersection Points/2(P32) -> Compute L2/5(P32)
  Compute L2/1(L2) -> L2 Vec/1

== system AutopilotControlSystem/GuidanceLogic/GuidanceLogic_Stateflow/GuidanceStateMachine/GuidanceLogic.Orbit/Minimum Turn Radius ==
  U_c : Inport
  Scale Factor : Inport  Port=2
  Constant1 : Constant  Value=ap.guidance.maxAcc  OutDataTypeStr=single
      settings: AttributesFormatString=%<Value>
  Math Function : Math  Operator=square  SaturateOnIntegerOverflow=on
  Product2 : Product  RndMeth=Zero
  Product3 : Product  Inputs=*/  RndMeth=Zero
  "[1.5 10]" : Saturate  UpperLimit=10  LowerLimit=1.5
      settings: AttributesFormatString="[%<LowerLimit>  %<UpperLimit>]"
  R : Outport  VectorParamsAs1DForOutWhenUnconnected=off
  wires:
  U_c/1 -> Math Function/1
  Product2/1 -> Product3/1
  Constant1/1 -> Product3/2
  Math Function/1 -> Product2/2
  Product3/1 -> R/1
  "[1.5 10]"/1 -> Product2/1
  Scale Factor/1 -> "[1.5 10]"/1

== system AutopilotControlSystem/GuidanceLogic/GuidanceLogic_Stateflow/GuidanceStateMachine/GuidanceLogic.Orbit/No intersection, Navigate to ISR ==
  Xe : Inport
  WP : Inport  Port=2
  Action Port : ActionPort  ActionPortLabel=if(u1 > u2)
  Subtract : Sum  Inputs=+-
  L2 Vec : Outport  VectorParamsAs1DForOutWhenUnconnected=off
  wires:
  Subtract/1 -> L2 Vec/1
  Xe/1 -> Subtract/2
  WP/1 -> Subtract/1

== system AutopilotControlSystem/GuidanceLogic/GuidanceLogic_Stateflow/GuidanceStateMachine/GuidanceLogic.RTB/Get Mobile Location ==
  Mobile Loc : Inport
  UAVMission : Inport  Port=2
  Enable : EnablePort
  Bus Selector1 : BusSelector  OutputSignals=wpPos
  Demux : Demux  Outputs=[2 1]
  LLA to Flat Earth : aerolibtransform2/LLA to Flat Earth  Commented=on  units=Metric (MKS)  ptype=Earth (WGS84)  F=1/298.257223563  R=6378137  LL0=[0 10]  psi=0
      settings: SourceProductName=Aerospace Blockset  SourceProductBaseCode=AE
  LLA to Flat Earth with Init Pos : mbdriLib/Coordinates/LLA to Flat Earth with Init Pos  R=6378137  F=1/298.2572235  psi=0
      settings: SourceProductName=Robotics System Toolbox  SourceProductBaseCode=RO
  Selector2 : Selector  InputPortWidth=10  IndexOptions=Index vector (dialog)  Indices=[1]  OutputSizes=1
  Selector3 : Selector  InputPortWidth=3  IndexOptions=Index vector (dialog)  Indices=[3]  OutputSizes=1
  Selector4 : Selector  InputPortWidth=3  IndexOptions=Index vector (dialog)  Indices=[1 2]  OutputSizes=1
  Subsystem3 : Subsystem
  MobileLTP : Outport  VectorParamsAs1DForOutWhenUnconnected=off
  wires:
  UAVMission/1 -> Selector2/1
  Demux/1 -> LLA to Flat Earth with Init Pos/1
  Selector3/1 -> LLA to Flat Earth with Init Pos/3
  Demux/2 -> LLA to Flat Earth with Init Pos/2
  Mobile Loc/1 -> Demux/1
  Selector2/1 -> Bus Selector1/1
  LLA to Flat Earth with Init Pos/1 -> Subsystem3/1("[a b c]")
  Selector4/1 -> LLA to Flat Earth with Init Pos/4
  Bus Selector1/1 -> Selector4/1, Selector3/1  "<wpPos>"
  Subsystem3/1("[a b 0]") -> MobileLTP/1

== system AutopilotControlSystem/GuidanceLogic/GuidanceLogic_Stateflow/GuidanceStateMachine/GuidanceLogic.RTB/Simple Predictor ==
  Base Point : Inport
  Prediction Gain : Inport  Port=2
  Discrete-Time Integrator : DiscreteIntegrator  InitialConditionSource=external  SampleTime=-1  ICPrevOutput=DiscIntNeverNeededParam  ICPrevScaledInput=DiscIntNeverNeededParam
  Product : Product  RndMeth=Zero
  Sum : Sum  Inputs=|+-
  Sum1 : Sum  Inputs=++|
  Predicted Bp : Outport  VectorParamsAs1DForOutWhenUnconnected=off
  wires:
  Sum/1 -> Discrete-Time Integrator/1, Product/2
  Discrete-Time Integrator/1 -> Sum/2, Sum1/2
  Product/1 -> Sum1/1
  Base Point/1 -> Sum/1, Discrete-Time Integrator/2
  Sum1/1 -> Predicted Bp/1
  Prediction Gain/1 -> Product/1

== system AutopilotControlSystem/GuidanceLogic/GuidanceLogic_Stateflow/GuidanceStateMachine/GuidanceLogic.WP/Compute Distance to WP ==
  Xe : Inport
  WPT : Inport  Port=2
  T : Inport  Port=3
  Dot Product : DotProduct  InputSameDT=on  OutDataTypeStr=Inherit: Inherit via internal rule
  Subtract : Sum  Inputs=-+  OutDataTypeStr=single
  Dist2WpT : Outport  VectorParamsAs1DForOutWhenUnconnected=off
  wires:
  T/1 -> Dot Product/2
  Subtract/1 -> Dot Product/1
  WPT/1 -> Subtract/2
  Xe/1 -> Subtract/1
  Dot Product/1 -> Dist2WpT/1

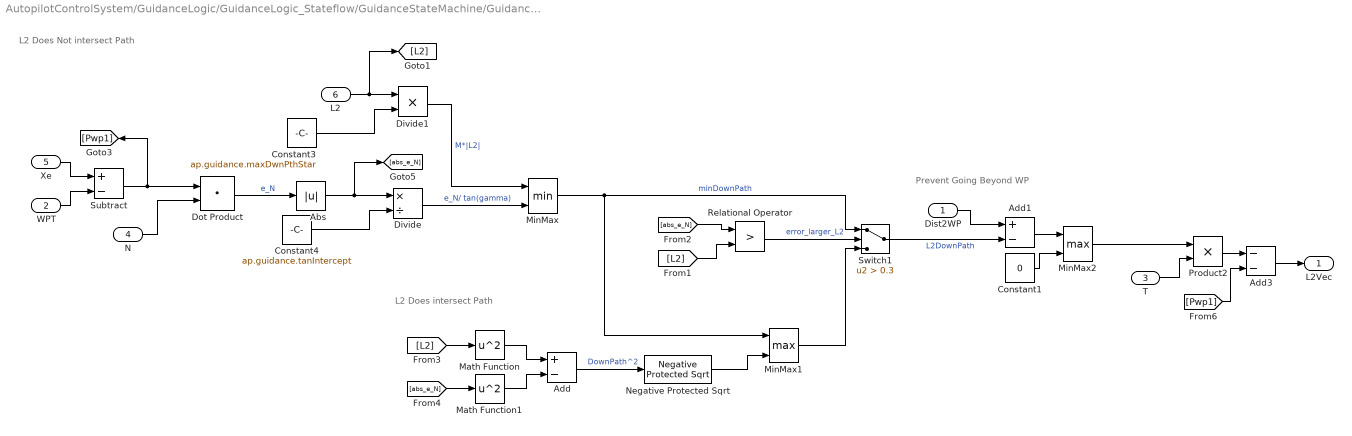
== system AutopilotControlSystem/GuidanceLogic/GuidanceLogic_Stateflow/GuidanceStateMachine/GuidanceLogic.WP/Compute L2 Vector ==
  note: Prevent Going Beyond WP
  note: L2 Does intersect Path
  note: L2 Does Not intersect Path
  Dist2WP : Inport
  WPT : Inport  Port=2
  T : Inport  Port=3
  N : Inport  Port=4
  Xe : Inport  Port=5
  L2 : Inport  Port=6
  Abs : Abs
  Add : Sum  Inputs=+-
  Add1 : Sum  Inputs=+-
  Add3 : Sum  Inputs=--
  Constant1 : Constant  Value=0  OutDataTypeStr=single
      settings: AttributesFormatString=%<Value>
  Constant3 : Constant  Value=ap.guidance.maxDwnPthStar  OutDataTypeStr=single
      settings: AttributesFormatString=%<Value>
  Constant4 : Constant  Value=ap.guidance.tanIntercept  OutDataTypeStr=single
      settings: AttributesFormatString=%<Value>
  Divide : Product  Inputs=*/
  Divide1 : Product
  Dot Product : DotProduct  InputSameDT=on  OutDataTypeStr=Inherit: Inherit via internal rule
  Math Function : Math  Operator=square  SaturateOnIntegerOverflow=on
  Math Function1 : Math  Operator=square  SaturateOnIntegerOverflow=on
  MinMax : MinMax  Inputs=2
  MinMax1 : MinMax  Function=max  Inputs=2
  MinMax2 : MinMax  Function=max  Inputs=2
  Negative Protected Sqrt : mbdriLib/Utilities/Negative Protected Sqrt  SystemSampleTime=-1  Latency=0  AutoFrameSizeCalculation=off
      settings: SourceProductName=Robotics System Toolbox  SourceProductBaseCode=RO
  Product2 : Product  RndMeth=Zero
  Relational Operator : RelationalOperator  Operator=>  OutDataTypeStr=boolean  RndMeth=Nearest
  Subtract : Sum  Inputs=+-  OutDataTypeStr=single
  Switch1 : Switch  Criteria=u2 > Threshold  Threshold=0.3
  L2Vec : Outport  VectorParamsAs1DForOutWhenUnconnected=off
  wires:
  Xe/1 -> Subtract/1
  WPT/1 -> Subtract/2
  Subtract/1 -> Dot Product/1, [Pwp1]
  Dot Product/1 -> Abs/1  "e_N"
  Abs/1 -> Divide/1, [abs_e_N]
  Constant4/1 -> Divide/2
  Divide/1 -> MinMax/2  "e_N/ tan(gamma)"
  L2/1 -> Divide1/1, [L2]
  Constant3/1 -> Divide1/2
  Divide1/1 -> MinMax/1  "M*|L2|"
  MinMax/1 -> MinMax1/1, Switch1/1  "minDownPath"
  Relational Operator/1 -> Switch1/2  "error_larger_L2"
  [L2] -> Relational Operator/2
  [abs_e_N] -> Relational Operator/1
  Switch1/1 -> Add1/2  "L2DownPath"
  Add/1 -> Negative Protected Sqrt/1  "DownPath^2"
  Negative Protected Sqrt/1 -> MinMax1/2
  [L2] -> Math Function/1
  Math Function/1 -> Add/1
  [abs_e_N] -> Math Function1/1
  Math Function1/1 -> Add/2
  MinMax1/1 -> Switch1/3
  Add1/1 -> MinMax2/1
  Constant1/1 -> MinMax2/2
  MinMax2/1 -> Product2/1
  T/1 -> Product2/2
  Product2/1 -> Add3/1
  [Pwp1] -> Add3/2
  Add3/1 -> L2Vec/1
  N/1 -> Dot Product/2
  Dist2WP/1 -> Add1/1

== system AutopilotControlSystem/GuidanceLogic/GuidanceLogic_Stateflow/GuidanceStateMachine/GuidanceLogic.WP/Compute Vg_norm ==
  <Ve_hat> : Inport
  " Compute Norm" : mbdriLib/Utilities/ Compute Norm  SystemSampleTime=-1  Latency=0  AutoFrameSizeCalculation=off
      settings: SourceProductName=Robotics System Toolbox  SourceProductBaseCode=RO
  Zero Out Z : mbdriLib/Utilities/Zero Out Z  SystemSampleTime=-1  Latency=0  AutoFrameSizeCalculation=off
      settings: SourceProductName=Robotics System Toolbox  SourceProductBaseCode=RO
  |Vg| : Outport  VectorParamsAs1DForOutWhenUnconnected=off
  wires:
  <Ve_hat>/1 -> Zero Out Z/1
  Zero Out Z/1 -> " Compute Norm"/1
  " Compute Norm"/1 -> |Vg|/1  "|Vg|"

== system AutopilotControlSystem/GuidanceLogic/GuidanceLogic_Stateflow/GuidanceStateMachine/GuidanceLogic.WP/Get Next Waypoint ==
  UAVMission : Inport
  From WP : Inport  Port=2
  To WP : Inport  Port=3
  L2 : Inport  Port=4
  Compute Frenet Frame : Subsystem
  Compute WPT : Subsystem  TreatAsAtomicUnit=on
  Selector : Selector  InputPortWidth=3  IndexOptions=Index vector (dialog)  Indices=[3]  OutputSizes=1
  Terminator : Terminator
  Zero Out Z : mbdriLib/Utilities/Zero Out Z  SystemSampleTime=-1  Latency=0  AutoFrameSizeCalculation=off
      settings: SourceProductName=Robotics System Toolbox  SourceProductBaseCode=RO
  Zero Out Z1 : mbdriLib/Utilities/Zero Out Z  SystemSampleTime=-1  Latency=0  AutoFrameSizeCalculation=off
      settings: SourceProductName=Robotics System Toolbox  SourceProductBaseCode=RO
  Zero Out Z2 : mbdriLib/Utilities/Zero Out Z  SystemSampleTime=-1  Latency=0  AutoFrameSizeCalculation=off
      settings: SourceProductName=Robotics System Toolbox  SourceProductBaseCode=RO
  H_c : Outport  VectorParamsAs1DForOutWhenUnconnected=off
  WPT : Outport  Port=2  VectorParamsAs1DForOutWhenUnconnected=off
  T : Outport  Port=3  VectorParamsAs1DForOutWhenUnconnected=off
  N : Outport  Port=4  VectorParamsAs1DForOutWhenUnconnected=off
  wires:
  From WP/1 -> Compute WPT/1(FromWP), Compute Frenet Frame/2(idx_F)
  To WP/1 -> Compute Frenet Frame/3(idx_T)
  Compute Frenet Frame/3(T) -> Zero Out Z1/1, Compute WPT/3(T)
  Compute Frenet Frame/4(N) -> Zero Out Z2/1
  Zero Out Z1/1 -> T/1
  Zero Out Z2/1 -> N/1
  UAVMission/1 -> Compute Frenet Frame/1(uavMission)
  Compute WPT/1(WPT_out) -> Zero Out Z/1, Selector/1
  Compute Frenet Frame/2(WPT) -> Compute WPT/2(WPT_in)
  L2/1 -> Compute WPT/4(L2)
  Zero Out Z/1 -> WPT/1
  Selector/1 -> H_c/1
  Compute Frenet Frame/1(WPF) -> Terminator/1

== system AutopilotControlSystem/GuidanceLogic/GuidanceLogic_Stateflow/GuidanceStateMachine/GuidanceLogic.WP/Recent Enable ==
  WP Fly : Inport
  Logical Operator : Logic  AllPortsSameDT=off  OutDataTypeStr=boolean
  Logical Operator1 : Logic  Operator=NOT  AllPortsSameDT=off  OutDataTypeStr=boolean
  Unit Delay : UnitDelay  SampleTime=-1  HasFrameUpgradeWarning=on
  WPEnable : Outport  VectorParamsAs1DForOutWhenUnconnected=off
  wires:
  Logical Operator/1 -> WPEnable/1
  Logical Operator1/1 -> Logical Operator/2
  Unit Delay/1 -> Logical Operator1/1
  WP Fly/1 -> Unit Delay/1, Logical Operator/1

== system AutopilotControlSystem/InnerLoopAutopilot/Longitudinal Channel/Rate Limiter Dynamic with External IC and Autoreset for Change in IC/Capture//Reset IC ==
  Y(k) : Inport
  IC : Inport  Port=2
  Abs : Abs
  Delay : Delay  DelayLength=1
  Subsystem : Subsystem
  Subtract : Sum  Inputs=+-
  Unit Delay Resettable External IC : simulink_need_slupdate/Unit Delay Resettable External IC  tsamp=-1
      settings: SourceProductName=Simulink  SourceProductBaseCode=SL
  Y(k-1) : Outport  VectorParamsAs1DForOutWhenUnconnected=off
  wires:
  Unit Delay Resettable External IC/1 -> Y(k-1)/1  "Y(k-1)"
  Y(k)/1 -> Unit Delay Resettable External IC/1
  Subtract/1 -> Abs/1
  Abs/1 -> Subsystem/1(WP Fly)
  IC/1 -> Delay/1, Subtract/2, Unit Delay Resettable External IC/3
  Subsystem/1(Just Enab) -> Unit Delay Resettable External IC/2
  Delay/1 -> Subtract/1

== system AutopilotControlSystem/GuidanceLogic/GuidanceLogic_Simulink/Guidance/Circle Guidance/Get WP Location ==
  viewPoint : Inport
  UAVMission : Inport  Port=2
  Bus Selector : BusSelector  OutputSignals=wpPos
  Bus Selector1 : BusSelector  OutputSignals=wpPos
  Demux : Demux  Outputs=[2 1]
  Integer Delay1 : Delay  DelayLength=1
  LLA to Flat Earth : aerolibtransform2/LLA to Flat Earth  Commented=on  units=Metric (MKS)  ptype=Earth (WGS84)  F=1/298.257223563  R=6378137  LL0=[0 10]  psi=0
      settings: SourceProductName=Aerospace Blockset  SourceProductBaseCode=AE
  LLA to Flat Earth with Init Pos : mbdriLib/Coordinates/LLA to Flat Earth with Init Pos  R=6378137  F=1/298.2572235  psi=0
      settings: SourceProductName=Robotics System Toolbox  SourceProductBaseCode=RO
  Selector : Selector  InputPortWidth=3  IndexOptions=Index vector (dialog)  Indices=[3]  OutputSizes=1
  Selector1 : Selector  InputPortWidth=10  IndexOptions=Index vector (port)  Indices=[3]  OutputSizes=1
  Selector2 : Selector  InputPortWidth=10  IndexOptions=Index vector (dialog)  Indices=[1]  OutputSizes=1
  Selector3 : Selector  InputPortWidth=3  IndexOptions=Index vector (dialog)  Indices=[3]  OutputSizes=1
  Selector4 : Selector  InputPortWidth=3  IndexOptions=Index vector (dialog)  Indices=[1 2]  OutputSizes=1
  Zero Out Z : mbdriLib/Utilities/Zero Out Z
      settings: SourceProductName=Robotics System Toolbox  SourceProductBaseCode=RO
  Hc : Outport  VectorParamsAs1DForOutWhenUnconnected=off
  WP : Outport  Port=2  VectorParamsAs1DForOutWhenUnconnected=off
  wires:
  Zero Out Z/1 -> WP/1
  LLA to Flat Earth with Init Pos/1 -> Zero Out Z/1, Selector/1
  Selector4/1 -> LLA to Flat Earth with Init Pos/4
  Selector2/1 -> Bus Selector1/1
  Selector3/1 -> LLA to Flat Earth with Init Pos/3
  Demux/1 -> LLA to Flat Earth with Init Pos/1
  Demux/2 -> LLA to Flat Earth with Init Pos/2
  Bus Selector/1 -> Demux/1  "<wpPos>"
  Selector1/1 -> Bus Selector/1
  viewPoint/1 -> Selector1/2
  UAVMission/1 -> Selector1/1, Selector2/1
  Integer Delay1/1 -> Hc/1
  Selector/1 -> Integer Delay1/1
  Bus Selector1/1 -> Selector4/1, Selector3/1  "<wpPos>"

== system AutopilotControlSystem/GuidanceLogic/GuidanceLogic_Simulink/Guidance/Circle Guidance/Inside the Circle, Keep Straight until intersection ==
  note: % Compute the top coordinate of the circle
      | % using the circle's parametric equations:
      | % x = a + r cos (t)
      | % y = b + r sin (t)
      | %
      | % @ t =0
  WP : Inport
  R : Inport  Port=2
  Xe : Inport  Port=3
  Action Port : ActionPort  ActionPortLabel=elseif { }
  Demux : Demux  Outputs=[1 2]
  Mux : Mux  Inputs=2
  Subtract : Sum  Inputs=+-  OutDataTypeStr=single
  Subtract1 : Sum  OutDataTypeStr=single
  L2 Vec : Outport  VectorParamsAs1DForOutWhenUnconnected=off
  wires:
  Mux/1 -> Subtract/1
  WP/1 -> Demux/1
  R/1 -> Subtract1/1
  Demux/2 -> Mux/2
  Subtract1/1 -> Mux/1
  Demux/1 -> Subtract1/2
  Xe/1 -> Subtract/2
  Subtract/1 -> L2 Vec/1

== system AutopilotControlSystem/GuidanceLogic/GuidanceLogic_Simulink/Guidance/Circle Guidance/Intersection. Circular Navigation ==
  R : Inport
  L2 : Inport  Port=2
  d : Inport  Port=3
  WP : Inport  Port=4
  Ve : Inport  Port=5
  |Vg| : Inport  Port=6
  Xe : Inport  Port=7
  Action Port : ActionPort  ActionPortLabel=else { }
  Compute Hyp : Subsystem
  Compute L2 : Subsystem
  Compute P2 : Subsystem
  Compute the Intersection Points : MATLAB Function  TreatAsAtomicUnit=on
  Product5 : Product  RndMeth=Zero
  Xe1 : InportShadow  Port=7
  "d " : InportShadow  Port=3
  L2 Vec : Outport  VectorParamsAs1DForOutWhenUnconnected=off
  wires:
  Compute L2/1(L2) -> L2 Vec/1
  Compute the Intersection Points/2(P32) -> Compute L2/5(P32)
  Xe/1 -> Compute L2/4(Xe)
  Compute the Intersection Points/1(P31) -> Compute L2/3(P31)
  |Vg|/1 -> Compute L2/2(|Vg|)
  Ve/1 -> Compute L2/1(Ve)
  Compute P2/2(P2) -> Compute the Intersection Points/2(P2)
  Compute P2/1((Xe-Wp)/d) -> Product5/2
  Xe1/1 -> Compute P2/4(Xe)
  WP/1 -> Compute P2/3(WP)
  "d "/1 -> Compute P2/2(d)
  Compute Hyp/2(a) -> Compute P2/1(a)
  Compute Hyp/1(h) -> Product5/1
  d/1 -> Compute Hyp/3(d)
  L2/1 -> Compute Hyp/2(L2)
  R/1 -> Compute Hyp/1(R)
  Product5/1 -> Compute the Intersection Points/1(hFact)

== system AutopilotControlSystem/GuidanceLogic/GuidanceLogic_Simulink/Guidance/Circle Guidance/No intersection, Navigate to ISR ==
  Xe : Inport
  WP : Inport  Port=2
  Action Port : ActionPort  ActionPortLabel=if { }
  Subtract : Sum  Inputs=+-
  L2 Vec : Outport  VectorParamsAs1DForOutWhenUnconnected=off
  wires:
  WP/1 -> Subtract/1
  Xe/1 -> Subtract/2
  Subtract/1 -> L2 Vec/1
